simulink model "g729_encoder_verilog_test"  (Simulink 8.1)
settings: Solver=ode45  StartTime=0.0  StopTime=80000  RelTol=1e-3
libraries: xbsIndex_r4 x10
settings Model: Creator=aruls  LastModifiedBy=aruls
settings DataIOCC: SignalLoggingSaveFormat=Dataset
settings OptimizationCC: ExpressionDepthLimit=128
settings DebuggingCC: FcnCallInpInsideContextMsg=EnableAllAsError
settings GRTTargetCC: CombineOutputUpdateFcns=on  GRTInterface=off

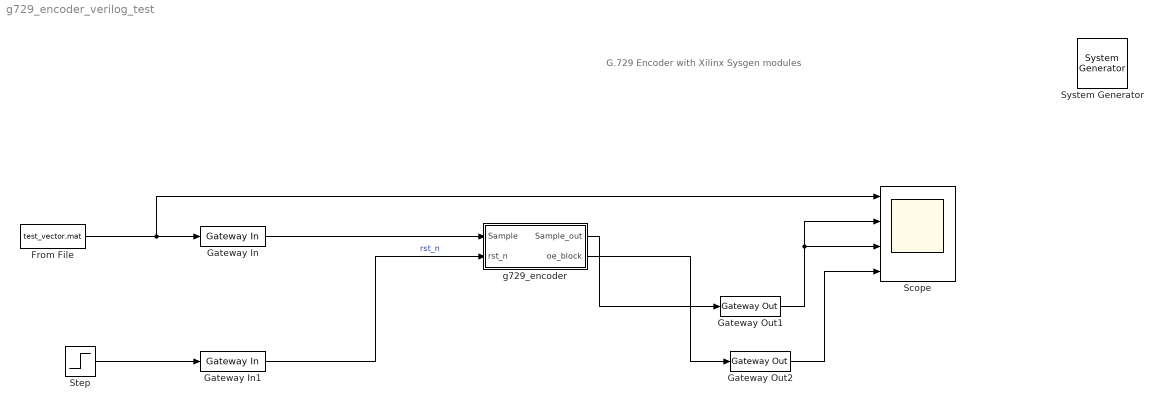
== system g729_encoder_verilog_test ==
  note: G.729 Encoder with Xilinx Sysgen modules
  " System Generator" : xbsIndex_r4/ System Generator  Tag=genX  xilinxfamily=spartan6  part=xc6slx100  speed=-3  package=fgg484  synthesis_tool=XST  clock_wrapper=Clock Enables  directory=./ngc_netlist  proj_type=Project Navigator  Synth_file=XST Defaults  Impl_file=ISE Defaults  testbench=off  simulink_period=1  sysclk_period=15.625  dcm_input_clock_period=10  incr_netlist=off  trim_vbits=Everywhere in SubSystem  dbl_ovrd=According to Block Masks  core_generation=According to Block Masks  run_coregen=off  deprecated_control=off  eval_field=0  block_type=sysgen
  From File : FromFile  FileName=test_vector.mat  SampleTime=10
  Gateway In : xbsIndex_r4/Gateway In  gui_display_data_type=Floating-point  arith_type=Floating-point  n_bits=16  bin_pt=14  preci_type=Single  exp_width=8  frac_width=24  quantization="Round  (unbiased: +/- Inf)"  overflow=Saturate  period=1  dbl_ovrd=off  timing_constraint=None  locs_specified=off  LOCs={}  UseAsADC=off  ADCChannel='1'  inherit_from_input=off  hdl_port=on  block_type=gatewayin
  Gateway In1 : xbsIndex_r4/Gateway In  gui_display_data_type=Boolean  arith_type=Boolean  n_bits=1  bin_pt=0  preci_type=Single  exp_width=8  frac_width=24  quantization="Round  (unbiased: +/- Inf)"  overflow=Saturate  period=1  dbl_ovrd=off  timing_constraint=None  locs_specified=off  LOCs={}  UseAsADC=off  ADCChannel='1'  inherit_from_input=off  hdl_port=on  block_type=gatewayin
  Gateway Out1 : xbsIndex_r4/Gateway Out  inherit_from_input=on  hdl_port=on  timing_constraint=None  locs_specified=off  LOCs={}  UseAsDAC=off  DACChannel='1'  block_type=gatewayout
  Gateway Out2 : xbsIndex_r4/Gateway Out  inherit_from_input=off  hdl_port=on  timing_constraint=None  locs_specified=off  LOCs={}  UseAsDAC=off  DACChannel='1'  block_type=gatewayout
  Scope : Scope  NumInputPorts=4
      settings: TimeRange=80000  YMin=-0.05~-0.02~-0.02~0  YMax=0.05~0.025~0.025~1.5e-42  MaxDataPoints=80000
  Step : Step  SampleTime=0
  g729_encoder : Subsystem
  wires:
  Gateway In1/1 -> g729_encoder/2(rst_n)  "rst_n"
  Step/1 -> Gateway In1/1
  From File/1 -> Gateway In/1, Scope/1
  Gateway Out1/1 -> Scope/2, Scope/3
  g729_encoder/1(Sample_out) -> Gateway Out1/1
  g729_encoder/2(oe_block) -> Gateway Out2/1
  Gateway Out2/1 -> Scope/4
  Gateway In/1 -> g729_encoder/1(Sample)

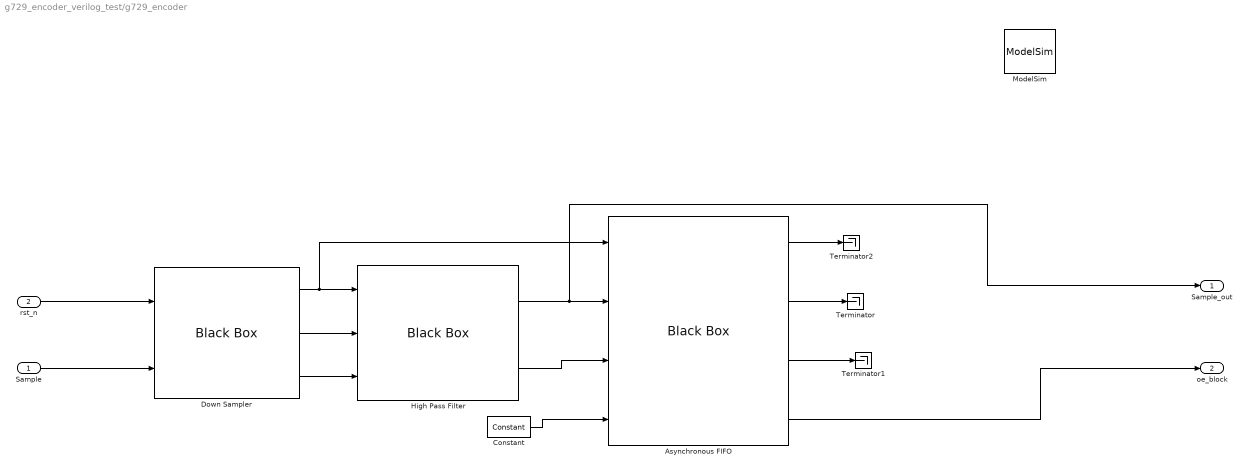
== system g729_encoder_verilog_test/g729_encoder ==
  Sample : Inport
  rst_n : Inport  Port=2
  Asynchronous FIFO : xbsIndex_r4/Black Box  init_code=ads_async_fifo_config  sim_method=External co-simulator  engine_block=ModelSim  verbose=off  block_type=blackbox2
  Constant : xbsIndex_r4/Constant  const=1  gui_display_data_type=Boolean  arith_type=Boolean  n_bits=16  bin_pt=14  preci_type=Single  exp_width=8  frac_width=24  explicit_period=off  period=1  equ=P=C  opselect=C  inp2=PCIN>>17  opr=+  inp1=P  carry=CIN  dbl_ovrd=off  block_type=constant
  Down Sampler : xbsIndex_r4/Black Box  init_code=dwn_sampler_config  sim_method=External co-simulator  engine_block=ModelSim  verbose=off  block_type=blackbox2
  High Pass Filter : xbsIndex_r4/Black Box  init_code=hpf_filter_config  sim_method=External co-simulator  engine_block=ModelSim  verbose=off  block_type=blackbox2
  ModelSim : xbsIndex_r4/ModelSim  dir=./modelsim  waveform=on  leave_open=on  skip_compile=off  use_unisim=on  use_ver_xilinxcorelib=on  custom_scripts=on  post_vsim_script=my.do  startup_timeout=40  block_type=hdlcosim
      settings: infoedit="Allow other blocks to schedule HDL co-simulation tasks.<br><br>Note that selecting \"Skip compilation\" when inappropriate can cause simulation errors and failures. Please refer to the block help for details."
  Terminator : Terminator
  Terminator1 : Terminator
  Terminator2 : Terminator
  Sample_out : Outport
  oe_block : Outport  Port=2
  wires:
  rst_n/1 -> Down Sampler/1
  Sample/1 -> Down Sampler/2
  Down Sampler/1 -> Asynchronous FIFO/1, High Pass Filter/1
  Down Sampler/3 -> High Pass Filter/3
  Down Sampler/2 -> High Pass Filter/2
  High Pass Filter/2 -> Asynchronous FIFO/3
  Asynchronous FIFO/2 -> Terminator/1
  Constant/1 -> Asynchronous FIFO/4
  Asynchronous FIFO/3 -> Terminator1/1
  High Pass Filter/1 -> Sample_out/1, Asynchronous FIFO/2
  Asynchronous FIFO/1 -> Terminator2/1
  Asynchronous FIFO/4 -> oe_block/1
